simulink model "PHIL_DHS_XY_Control"  (R2019b)
settings: Solver=VariableStepAuto  StartTime=0.0  StopTime=00.2  RelTol=1e-3
undefined symbols (not defined in the file): Apd_i_dhs, Apd_u_dhs, C_dhs, f_sw_dhs, L_dhs, L_drom, Tid_i_dhs, Tid_u_dhs, U_DC
libraries: coordinate_transformations x9, simulink x8
settings Model: Creator=kissd  LastModifiedBy=kissd

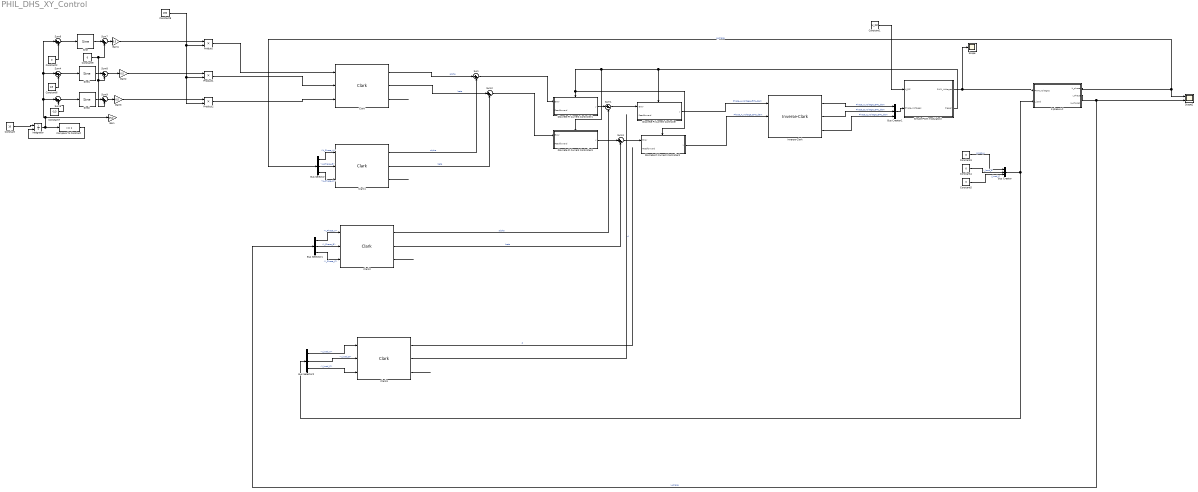
== system PHIL_DHS_XY_Control ==
  3 phase LC : Subsystem
  Bus Creator : BusCreator  Inputs=3
  Bus Creator1 : BusCreator  Inputs=3
  Bus Selector : BusSelector  OutputSignals=U_Phase_A,U_Phase_B,U_Phase_C
  Bus Selector1 : BusSelector  OutputSignals=I_Phase_A,I_Phase_B,I_Phase_C
  Bus Selector2 : BusSelector  OutputSignals=I_load_A,I_load_B,I_load_C
  Clark{,1..3} (4 alike) : coordinate_transformations/Clark  SystemSampleTime=-1  Latency=0  AutoFrameSizeCalculation=off
  Compare To Constant : simulink/Logic and Bit Operations/Compare To Constant  relop=>=  const=1  OutDataTypeStr=boolean
  Constant : Constant  Value=10
  Constant1 : Constant  Value=U_DC
  Constant{2..5,9} (5 alike) : Constant  Value=0
  Constant6 : Constant  Value=1/3
  Constant7 : Constant  Value=-1/3
  Constant8 : Constant  Value=200
  Discrete PI Current Controller : Subsystem  AncestorBlock=controllers/Discrete PI Controller  mask(Continous PI Controller){Apd=Apd_i_dhs, Tid=Tid_i_dhs, fs=f_sw_dhs, UpperSat=U_DC, LowerSat=0}
      mask prompts: Apd "Proprotional Gain"; Tid "Integration Time"; fs "fsw"; UpperSat "Max. Saturation"; LowerSat "Min. Saturation"
      mask help: Continous PI Controller description.
  Discrete PI Current Controller1 : Subsystem  AncestorBlock=controllers/Discrete PI Controller  mask(Continous PI Controller){Apd=Apd_u_dhs, Tid=Tid_u_dhs, fs=f_sw_dhs, UpperSat=200, LowerSat=-200}
      mask prompts: Apd "Proprotional Gain"; Tid "Integration Time"; fs "fsw"; UpperSat "Max. Saturation"; LowerSat "Min. Saturation"
      mask help: Continous PI Controller description.
  Discrete PI Current Controller2 : Subsystem  AncestorBlock=controllers/Discrete PI Controller  mask(Continous PI Controller){Apd=Apd_i_dhs, Tid=Tid_i_dhs, fs=f_sw_dhs, UpperSat=U_DC, LowerSat=0}
      mask prompts: Apd "Proprotional Gain"; Tid "Integration Time"; fs "fsw"; UpperSat "Max. Saturation"; LowerSat "Min. Saturation"
      mask help: Continous PI Controller description.
  Discrete PI Current Controller3 : Subsystem  AncestorBlock=controllers/Discrete PI Controller  mask(Continous PI Controller){Apd=Apd_u_dhs, Tid=Tid_u_dhs, fs=f_sw_dhs, UpperSat=200, LowerSat=-200}
      mask prompts: Apd "Proprotional Gain"; Tid "Integration Time"; fs "fsw"; UpperSat "Max. Saturation"; LowerSat "Min. Saturation"
      mask help: Continous PI Controller description.
  Gain : Gain  Gain=2*pi
  Gain1 : Gain  Gain=0.5
  Gain2 : Gain  Gain=0.5
  Gain3 : Gain  Gain=0.5
  Integrator : Integrator  ExternalReset=either
  Inverse-Clark : coordinate_transformations/Inverse-Clark  SystemSampleTime=-1  Latency=0  AutoFrameSizeCalculation=off
  Product : Product
  Product1 : Product
  Product2 : Product
  Scope : Scope
  Scope2 : Scope  NumInputPorts=2
  Simple PWM modulator2 : Subsystem  AncestorBlock=controllers/Simple PWM modulator
  Sine : simulink/Lookup Tables/Sine  Formula=sin(2*pi*u)  NumDataPoints=(2^5)+1  OutputWordLength=16  InternalRulePriority=Speed
      settings: SourceProductName=Simulink
  Sine1 : simulink/Lookup Tables/Sine  Formula=sin(2*pi*u)  NumDataPoints=(2^5)+1  OutputWordLength=16  InternalRulePriority=Speed
      settings: SourceProductName=Simulink
  Sine2 : simulink/Lookup Tables/Sine  Formula=sin(2*pi*u)  NumDataPoints=(2^5)+1  OutputWordLength=16  InternalRulePriority=Speed
      settings: SourceProductName=Simulink
  Sum{,1..3} (4 alike) : Sum  Inputs=|+-
  Sum{4..9} (6 alike) : Sum  Inputs=|++
  wires:
  Constant1/1 -> Simple PWM modulator2/1(U_DC)
  Inverse-Clark/3 -> Bus Creator1/3  "Phase_C_Voltage_EMU_dem"
  Inverse-Clark/2 -> Bus Creator1/2  "Phase_B_Voltage_EMU_dem"
  Sum1/1 -> Discrete PI Current Controller/1(Error)
  Inverse-Clark/1 -> Bus Creator1/1  "Phase_A_Voltage_EMU_dem"
  Simple PWM modulator2/1(PWM_Voltages) -> Scope/1, 3 phase LC/1(PWM_Voltages)
  Bus Creator1/1 -> Simple PWM modulator2/2(Phase_Voltages)
  Discrete PI Current Controller1/1(y) -> Sum1/1
  Sum/1 -> Discrete PI Current Controller1/1(Error)
  Clark/1 -> Sum/1  "alpha"
  Clark/2 -> Sum2/1  "beta"
  Clark/3 -> ?
  3 phase LC/2(I_Phase) -> Bus Selector1/1, Scope2/2  "I_phase"
  3 phase LC/1(U_phase) -> Scope2/1, Bus Selector/1  "U_phase"
  Constant3/1 -> Bus Creator/1  "I_load_A"
  Constant4/1 -> Bus Creator/2  "I_load_B"
  Constant5/1 -> Bus Creator/3  "I_load_C"
  Bus Creator/1 -> Bus Selector2/1, 3 phase LC/2(I_load)
  Discrete PI Current Controller/1(y) -> Inverse-Clark/1  "Phase_A_Voltage_EMU_dem"
  Sum2/1 -> Discrete PI Current Controller3/1(Error)
  Discrete PI Current Controller3/1(y) -> Sum3/1
  Sum3/1 -> Discrete PI Current Controller2/1(Error)
  Discrete PI Current Controller2/1(y) -> Inverse-Clark/2  "Phase_A_Voltage_EMU_dem"
  Clark1/3 -> ?
  Clark1/1 -> Sum/2  "alpha"
  Clark1/2 -> Sum2/2  "beta"
  Clark2/3 -> ?
  Bus Selector/1 -> Clark1/1  "<U_Phase_A>"
  Bus Selector/2 -> Clark1/2  "<U_Phase_B>"
  Bus Selector/3 -> Clark1/3  "<U_Phase_C>"
  Bus Selector1/1 -> Clark2/1  "<I_Phase_A>"
  Bus Selector1/2 -> Clark2/2  "<I_Phase_B>"
  Bus Selector1/3 -> Clark2/3  "<I_Phase_C>"
  Clark2/1 -> Sum1/2  "alpha"
  Clark2/2 -> Sum3/2  "beta"
  Bus Selector2/3 -> Clark3/3  "<I_load_C>"
  Bus Selector2/1 -> Clark3/1  "<I_load_A>"
  Clark3/3 -> ?
  Bus Selector2/2 -> Clark3/2  "<I_load_B>"
  Clark3/1 -> ?  "d"
  Clark3/2 -> ?  "d"
  Simple PWM modulator2/2(trigger) -> Discrete PI Current Controller2/Trigger, Discrete PI Current Controller1/Trigger, Discrete PI Current Controller3/Trigger, Discrete PI Current Controller/Trigger
  Sum4/1 -> Sine1/1
  Sum5/1 -> Sine2/1
  Sum6/1 -> Sine/1
  Constant/1 -> Integrator/1
  Compare To Constant/1 -> Integrator/2
  Constant2/1 -> Sum6/2
  Constant6/1 -> Sum4/2
  Constant7/1 -> Sum5/2
  Sine/1 -> Sum7/1
  Integrator/1 -> Gain/1, Sum5/1, Sum4/1, Sum6/1, Compare To Constant/1
  Constant8/1 -> Product2/2, Product1/2, Product/2
  Product/1 -> Clark/1
  Product1/1 -> Clark/2
  Product2/1 -> Clark/3
  Sine1/1 -> Sum8/1
  Sine2/1 -> Sum9/1
  Sum9/1 -> Gain3/1
  Sum8/1 -> Gain2/1
  Sum7/1 -> Gain1/1
  Constant9/1 -> Sum7/2, Sum8/2, Sum9/2
  Gain1/1 -> Product/1
  Gain2/1 -> Product1/1
  Gain3/1 -> Product2/1

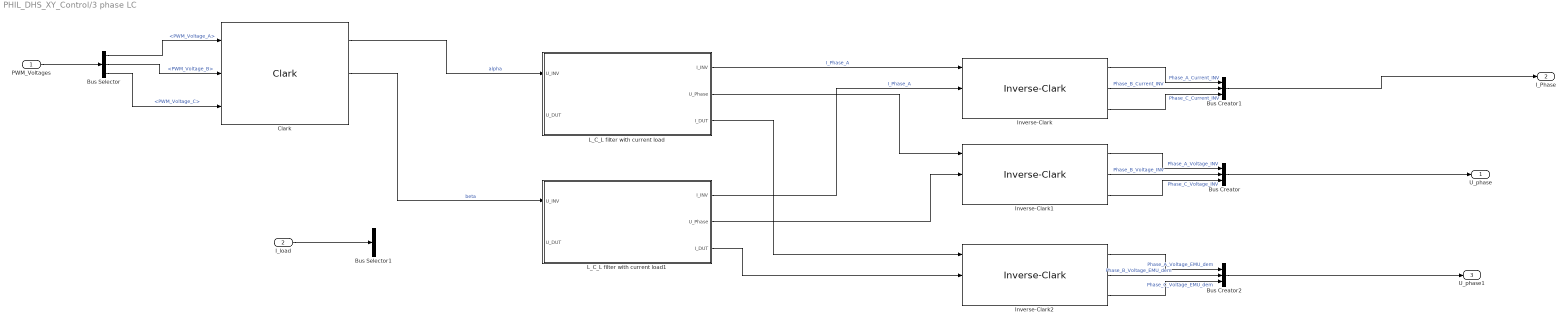
== system PHIL_DHS_XY_Control/3 phase LC ==
  PWM_Voltages : Inport
  I_load : Inport  Port=2
  Bus Creator : BusCreator  Inputs=3
  Bus Creator1 : BusCreator  Inputs=3
  Bus Creator2 : BusCreator  Inputs=3
  Bus Selector : BusSelector  OutputSignals=PWM_Voltage_A,PWM_Voltage_B,PWM_Voltage_C
  Bus Selector1 : BusSelector  OutputSignals=I_load_A,I_load_B,I_load_C
  Clark : coordinate_transformations/Clark  SystemSampleTime=-1  Latency=0  AutoFrameSizeCalculation=off
  Inverse-Clark : coordinate_transformations/Inverse-Clark  SystemSampleTime=-1  Latency=0  AutoFrameSizeCalculation=off
  Inverse-Clark1 : coordinate_transformations/Inverse-Clark  SystemSampleTime=-1  Latency=0  AutoFrameSizeCalculation=off
  Inverse-Clark2 : coordinate_transformations/Inverse-Clark  SystemSampleTime=-1  Latency=0  AutoFrameSizeCalculation=off
  L_C_L filter with current load : Subsystem
  L_C_L filter with current load1 : Subsystem
  U_phase : Outport
  I_Phase : Outport  Port=2
  U_phase1 : Outport  Port=3
  wires:
  PWM_Voltages/1 -> Bus Selector/1
  Bus Creator/1 -> U_phase/1
  Bus Creator1/1 -> I_Phase/1
  I_load/1 -> Bus Selector1/1
  Bus Selector/2 -> Clark/2  "<PWM_Voltage_B>"
  Bus Selector/1 -> Clark/1  "<PWM_Voltage_A>"
  Bus Selector/3 -> Clark/3  "<PWM_Voltage_C>"
  Clark/1 -> L_C_L filter with current load/1(U_INV)  "alpha"
  Clark/2 -> L_C_L filter with current load1/1(U_INV)  "beta"
  L_C_L filter with current load/1(I_INV) -> Inverse-Clark/1  "I_Phase_A"
  L_C_L filter with current load1/1(I_INV) -> Inverse-Clark/2  "I_Phase_A"
  L_C_L filter with current load/2(U_Phase) -> Inverse-Clark1/1
  L_C_L filter with current load1/2(U_Phase) -> Inverse-Clark1/2
  L_C_L filter with current load/3(I_DUT) -> Inverse-Clark2/1
  L_C_L filter with current load1/3(I_DUT) -> Inverse-Clark2/2
  Inverse-Clark1/2 -> Bus Creator/2  "Phase_B_Voltage_INV"
  Inverse-Clark1/1 -> Bus Creator/1  "Phase_A_Voltage_INV"
  Inverse-Clark1/3 -> Bus Creator/3  "Phase_C_Voltage_INV"
  Inverse-Clark/2 -> Bus Creator1/2  "Phase_B_Current_INV"
  Inverse-Clark/1 -> Bus Creator1/1  "Phase_A_Current_INV"
  Inverse-Clark/3 -> Bus Creator1/3  "Phase_C_Current_INV"
  Inverse-Clark2/1 -> Bus Creator2/1  "Phase_A_Voltage_EMU_dem"
  Inverse-Clark2/2 -> Bus Creator2/2  "Phase_B_Voltage_EMU_dem"
  Inverse-Clark2/3 -> Bus Creator2/3  "Phase_C_Voltage_EMU_dem"
  Bus Creator2/1 -> U_phase1/1

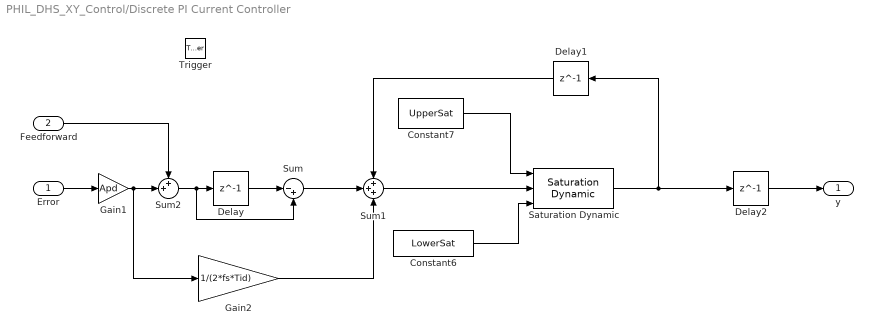
== system PHIL_DHS_XY_Control/Discrete PI Current Controller ==
  Error : Inport
  Feedforward : Inport  Port=2
  Trigger : TriggerPort  TriggerType=either  VariantControl=Variant  PortDimensions=1
  Constant6 : Constant  Value=LowerSat
  Constant7 : Constant  Value=UpperSat
  Delay : Delay  DelayLength=1
  Delay1 : Delay  DelayLength=1
  Delay2 : Delay  DelayLength=1
  Gain1 : Gain  Gain=Apd
  Gain2 : Gain  Gain=1/(2*fs*Tid)
  Saturation Dynamic : simulink/Discontinuities/Saturation Dynamic  OutMin=[]  OutMax=[]  OutDataTypeStr=Inherit: Same as second input  OutDataType=fixdt(1, 16)  OutScaling=2^-10  DoSatur=off
  Sum : Sum  Inputs=|-+
  Sum1 : Sum  Inputs=+++
  Sum2 : Sum  Inputs=++|
  y : Outport
  wires:
  Error/1 -> Gain1/1
  Gain1/1 -> Sum2/2, Gain2/1
  Sum1/1 -> Saturation Dynamic/2
  Saturation Dynamic/1 -> Delay1/1, Delay2/1
  Constant7/1 -> Saturation Dynamic/1
  Constant6/1 -> Saturation Dynamic/3
  Delay/1 -> Sum/1
  Sum/1 -> Sum1/2
  Gain2/1 -> Sum1/3
  Delay1/1 -> Sum1/1
  Delay2/1 -> y/1
  Sum2/1 -> Sum/2, Delay/1
  Feedforward/1 -> Sum2/1

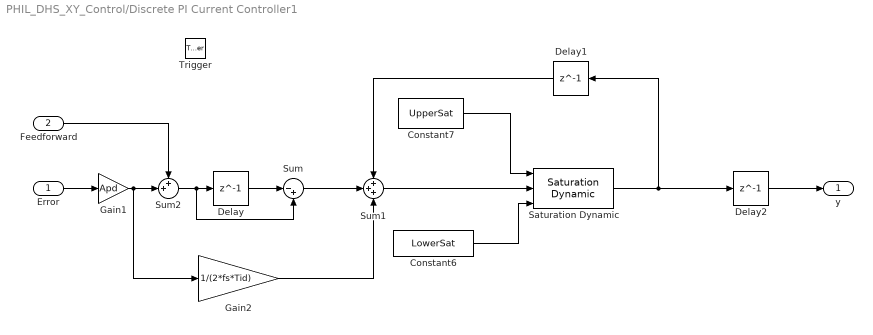
== system PHIL_DHS_XY_Control/Discrete PI Current Controller1 ==
  Error : Inport
  Feedforward : Inport  Port=2
  Trigger : TriggerPort  TriggerType=either  VariantControl=Variant  PortDimensions=1
  Constant6 : Constant  Value=LowerSat
  Constant7 : Constant  Value=UpperSat
  Delay : Delay  DelayLength=1
  Delay1 : Delay  DelayLength=1
  Delay2 : Delay  DelayLength=1
  Gain1 : Gain  Gain=Apd
  Gain2 : Gain  Gain=1/(2*fs*Tid)
  Saturation Dynamic : simulink/Discontinuities/Saturation Dynamic  OutMin=[]  OutMax=[]  OutDataTypeStr=Inherit: Same as second input  OutDataType=fixdt(1, 16)  OutScaling=2^-10  DoSatur=off
  Sum : Sum  Inputs=|-+
  Sum1 : Sum  Inputs=+++
  Sum2 : Sum  Inputs=++|
  y : Outport
  wires:
  Error/1 -> Gain1/1
  Gain1/1 -> Sum2/2, Gain2/1
  Sum1/1 -> Saturation Dynamic/2
  Saturation Dynamic/1 -> Delay1/1, Delay2/1
  Constant7/1 -> Saturation Dynamic/1
  Constant6/1 -> Saturation Dynamic/3
  Delay/1 -> Sum/1
  Sum/1 -> Sum1/2
  Gain2/1 -> Sum1/3
  Delay1/1 -> Sum1/1
  Delay2/1 -> y/1
  Sum2/1 -> Sum/2, Delay/1
  Feedforward/1 -> Sum2/1

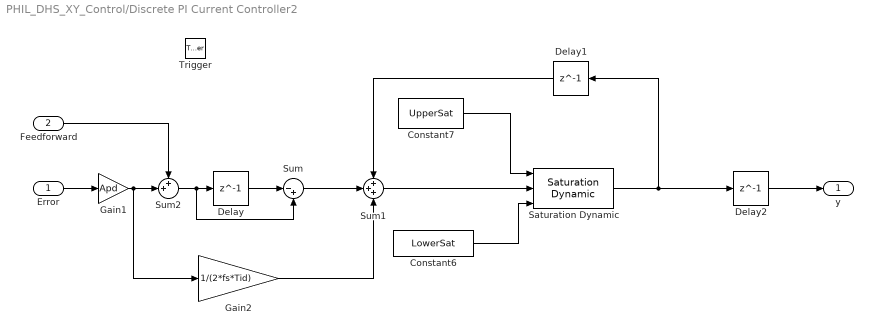
== system PHIL_DHS_XY_Control/Discrete PI Current Controller2 ==
  Error : Inport
  Feedforward : Inport  Port=2
  Trigger : TriggerPort  TriggerType=either  VariantControl=Variant  PortDimensions=1
  Constant6 : Constant  Value=LowerSat
  Constant7 : Constant  Value=UpperSat
  Delay : Delay  DelayLength=1
  Delay1 : Delay  DelayLength=1
  Delay2 : Delay  DelayLength=1
  Gain1 : Gain  Gain=Apd
  Gain2 : Gain  Gain=1/(2*fs*Tid)
  Saturation Dynamic : simulink/Discontinuities/Saturation Dynamic  OutMin=[]  OutMax=[]  OutDataTypeStr=Inherit: Same as second input  OutDataType=fixdt(1, 16)  OutScaling=2^-10  DoSatur=off
  Sum : Sum  Inputs=|-+
  Sum1 : Sum  Inputs=+++
  Sum2 : Sum  Inputs=++|
  y : Outport
  wires:
  Error/1 -> Gain1/1
  Gain1/1 -> Sum2/2, Gain2/1
  Sum1/1 -> Saturation Dynamic/2
  Saturation Dynamic/1 -> Delay1/1, Delay2/1
  Constant7/1 -> Saturation Dynamic/1
  Constant6/1 -> Saturation Dynamic/3
  Delay/1 -> Sum/1
  Sum/1 -> Sum1/2
  Gain2/1 -> Sum1/3
  Delay1/1 -> Sum1/1
  Delay2/1 -> y/1
  Sum2/1 -> Sum/2, Delay/1
  Feedforward/1 -> Sum2/1

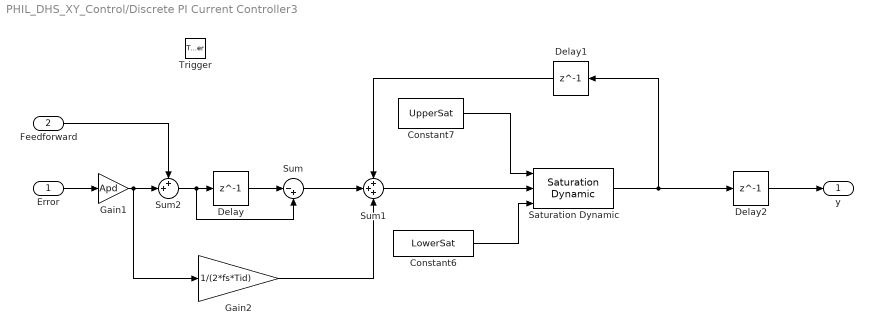
== system PHIL_DHS_XY_Control/Discrete PI Current Controller3 ==
  Error : Inport
  Feedforward : Inport  Port=2
  Trigger : TriggerPort  TriggerType=either  VariantControl=Variant  PortDimensions=1
  Constant6 : Constant  Value=LowerSat
  Constant7 : Constant  Value=UpperSat
  Delay : Delay  DelayLength=1
  Delay1 : Delay  DelayLength=1
  Delay2 : Delay  DelayLength=1
  Gain1 : Gain  Gain=Apd
  Gain2 : Gain  Gain=1/(2*fs*Tid)
  Saturation Dynamic : simulink/Discontinuities/Saturation Dynamic  OutMin=[]  OutMax=[]  OutDataTypeStr=Inherit: Same as second input  OutDataType=fixdt(1, 16)  OutScaling=2^-10  DoSatur=off
  Sum : Sum  Inputs=|-+
  Sum1 : Sum  Inputs=+++
  Sum2 : Sum  Inputs=++|
  y : Outport
  wires:
  Error/1 -> Gain1/1
  Gain1/1 -> Sum2/2, Gain2/1
  Sum1/1 -> Saturation Dynamic/2
  Saturation Dynamic/1 -> Delay1/1, Delay2/1
  Constant7/1 -> Saturation Dynamic/1
  Constant6/1 -> Saturation Dynamic/3
  Delay/1 -> Sum/1
  Sum/1 -> Sum1/2
  Gain2/1 -> Sum1/3
  Delay1/1 -> Sum1/1
  Delay2/1 -> y/1
  Sum2/1 -> Sum/2, Delay/1
  Feedforward/1 -> Sum2/1

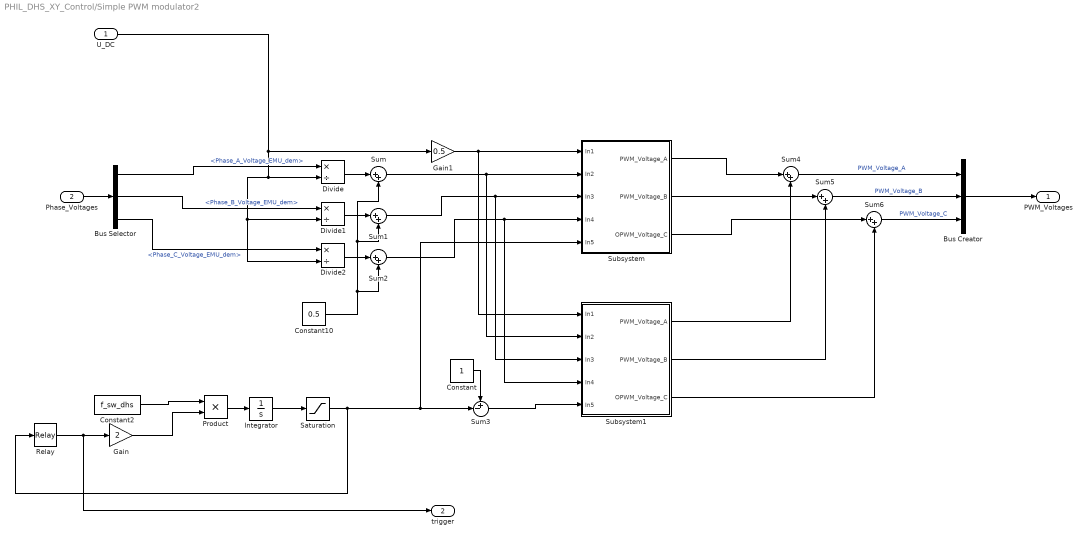
== system PHIL_DHS_XY_Control/Simple PWM modulator2 ==
  U_DC : Inport
  Phase_Voltages : Inport  Port=2
  Bus Creator : BusCreator  Inputs=3
  Bus Selector : BusSelector  OutputSignals=Phase_A_Voltage_EMU_dem,Phase_B_Voltage_EMU_dem,Phase_C_Voltage_EMU_dem
  Constant : Constant
  Constant10 : Constant  Value=0.5
  Constant2 : Constant  Value=f_sw_dhs
  Divide : Product  Inputs=*/
  Divide1 : Product  Inputs=*/
  Divide2 : Product  Inputs=*/
  Gain : Gain  Gain=2
  Gain1 : Gain  Gain=0.5
  Integrator : Integrator
  Product : Product
  Relay : Relay  OnSwitchValue=1  OffSwitchValue=0  OnOutputValue=-1  OffOutputValue=1
  Saturation : Saturate  UpperLimit=1  LowerLimit=0
  Subsystem : Subsystem
  Subsystem1 : Subsystem
  Sum{,1..2,4..6} (6 alike) : Sum  Inputs=|++
  Sum3 : Sum  Inputs=+-|
  PWM_Voltages : Outport
  trigger : Outport  Port=2
  wires:
  Constant2/1 -> Product/1
  Product/1 -> Integrator/1
  Integrator/1 -> Saturation/1
  Divide1/1 -> Sum1/1
  Saturation/1 -> Subsystem/5(In5), Sum3/2, Relay/1
  Relay/1 -> trigger/1, Gain/1
  Constant10/1 -> Sum2/2, Sum1/2, Sum/2
  Bus Selector/1 -> Divide/1  "<Phase_A_Voltage_EMU_dem>"
  Gain/1 -> Product/2
  Divide2/1 -> Sum2/1
  Divide/1 -> Sum/1
  Bus Selector/3 -> Divide2/1  "<Phase_C_Voltage_EMU_dem>"
  Bus Selector/2 -> Divide1/1  "<Phase_B_Voltage_EMU_dem>"
  Phase_Voltages/1 -> Bus Selector/1
  Bus Creator/1 -> PWM_Voltages/1
  Constant/1 -> Sum3/1
  Sum/1 -> Subsystem1/2(In2), Subsystem/2(In2)
  Sum1/1 -> Subsystem1/3(In3), Subsystem/3(In3)
  Sum2/1 -> Subsystem1/4(In4), Subsystem/4(In4)
  Sum3/1 -> Subsystem1/5(In5)
  Sum4/1 -> Bus Creator/1  "PWM_Voltage_A"
  Subsystem/1(PWM_Voltage_A) -> Sum4/1
  Subsystem1/1(PWM_Voltage_A) -> Sum4/2
  Sum5/1 -> Bus Creator/2  "PWM_Voltage_B"
  Subsystem/2(PWM_Voltage_B) -> Sum5/1
  Subsystem1/2(PWM_Voltage_B) -> Sum5/2
  Sum6/1 -> Bus Creator/3  "PWM_Voltage_C"
  Subsystem/3(OPWM_Voltage_C) -> Sum6/1
  Subsystem1/3(OPWM_Voltage_C) -> Sum6/2
  U_DC/1 -> Gain1/1, Divide2/2, Divide1/2, Divide/2
  Gain1/1 -> Subsystem1/1(In1), Subsystem/1(In1)

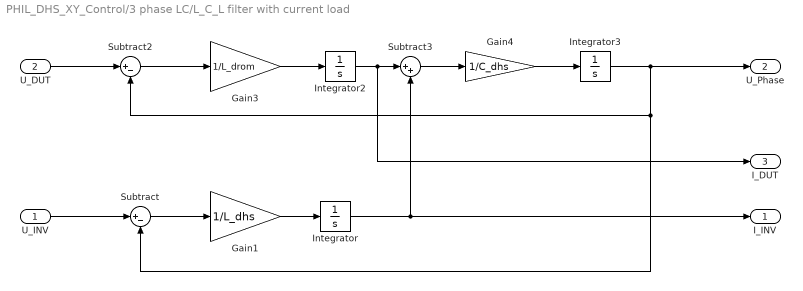
== system PHIL_DHS_XY_Control/3 phase LC/L_C_L filter with current load ==
  U_INV : Inport
  U_DUT : Inport  Port=2
  Gain1 : Gain  Gain=1/L_dhs
  Gain3 : Gain  Gain=1/L_drom
  Gain4 : Gain  Gain=1/C_dhs
  Integrator : Integrator
  Integrator2 : Integrator
  Integrator3 : Integrator
  Subtract : Sum  Inputs=|+-
  Subtract2 : Sum  Inputs=|+-
  Subtract3 : Sum  Inputs=|++
  I_INV : Outport
  U_Phase : Outport  Port=2
  I_DUT : Outport  Port=3
  wires:
  Subtract/1 -> Gain1/1
  Gain1/1 -> Integrator/1
  Integrator/1 -> Subtract3/2, I_INV/1
  U_INV/1 -> Subtract/1
  U_DUT/1 -> Subtract2/1
  Subtract2/1 -> Gain3/1
  Gain3/1 -> Integrator2/1
  Integrator2/1 -> I_DUT/1, Subtract3/1
  Subtract3/1 -> Gain4/1
  Gain4/1 -> Integrator3/1
  Integrator3/1 -> Subtract2/2, Subtract/2, U_Phase/1

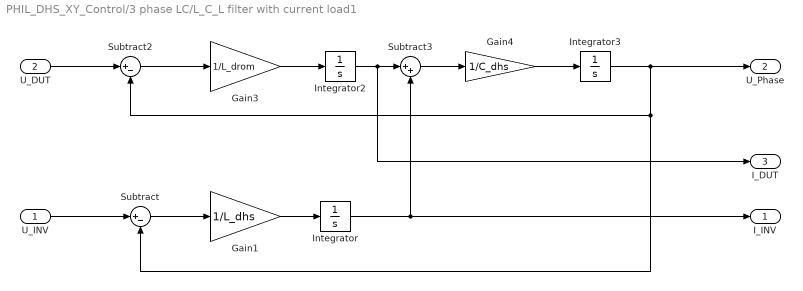
== system PHIL_DHS_XY_Control/3 phase LC/L_C_L filter with current load1 ==
  U_INV : Inport
  U_DUT : Inport  Port=2
  Gain1 : Gain  Gain=1/L_dhs
  Gain3 : Gain  Gain=1/L_drom
  Gain4 : Gain  Gain=1/C_dhs
  Integrator : Integrator
  Integrator2 : Integrator
  Integrator3 : Integrator
  Subtract : Sum  Inputs=|+-
  Subtract2 : Sum  Inputs=|+-
  Subtract3 : Sum  Inputs=|++
  I_INV : Outport
  U_Phase : Outport  Port=2
  I_DUT : Outport  Port=3
  wires:
  Subtract/1 -> Gain1/1
  Gain1/1 -> Integrator/1
  Integrator/1 -> Subtract3/2, I_INV/1
  U_INV/1 -> Subtract/1
  U_DUT/1 -> Subtract2/1
  Subtract2/1 -> Gain3/1
  Gain3/1 -> Integrator2/1
  Integrator2/1 -> I_DUT/1, Subtract3/1
  Subtract3/1 -> Gain4/1
  Gain4/1 -> Integrator3/1
  Integrator3/1 -> Subtract2/2, Subtract/2, U_Phase/1

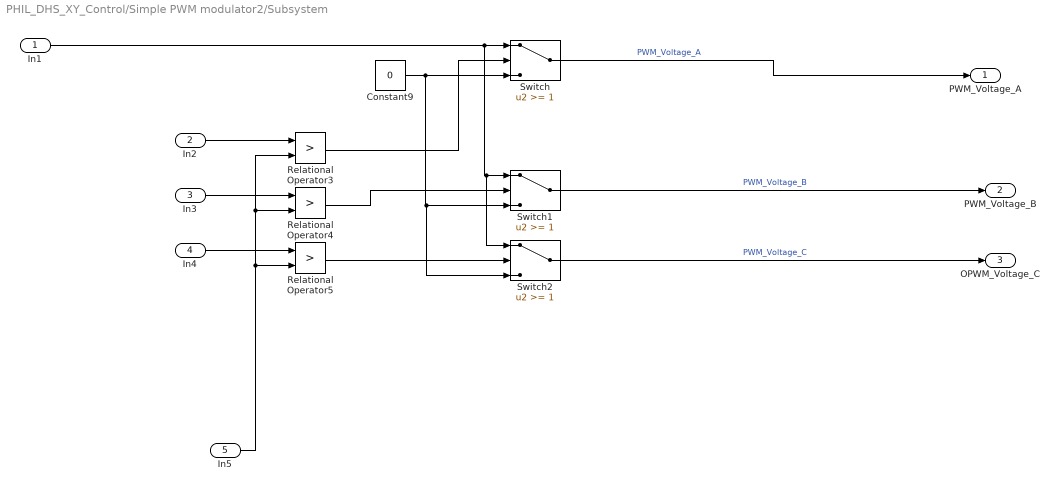
== system PHIL_DHS_XY_Control/Simple PWM modulator2/Subsystem ==
  In1 : Inport
  In2 : Inport  Port=2
  In3 : Inport  Port=3
  In4 : Inport  Port=4
  In5 : Inport  Port=5
  Constant9 : Constant  Value=0
  Relational Operator3 : RelationalOperator  Operator=>  OutDataTypeStr=boolean  RndMeth=Simplest
  Relational Operator4 : RelationalOperator  Operator=>  OutDataTypeStr=boolean  RndMeth=Simplest
  Relational Operator5 : RelationalOperator  Operator=>  OutDataTypeStr=boolean  RndMeth=Simplest
  Switch : Switch  Threshold=1
  Switch1 : Switch  Threshold=1
  Switch2 : Switch  Threshold=1
  PWM_Voltage_A : Outport
  PWM_Voltage_B : Outport  Port=2
  OPWM_Voltage_C : Outport  Port=3
  wires:
  Relational Operator4/1 -> Switch1/2
  In5/1 -> Relational Operator3/2, Relational Operator4/2, Relational Operator5/2
  Constant9/1 -> Switch2/3, Switch1/3, Switch/3
  Relational Operator3/1 -> Switch/2
  In3/1 -> Relational Operator4/1
  Relational Operator5/1 -> Switch2/2
  Switch/1 -> PWM_Voltage_A/1  "PWM_Voltage_A"
  In1/1 -> Switch2/1, Switch1/1, Switch/1
  In2/1 -> Relational Operator3/1
  In4/1 -> Relational Operator5/1
  Switch1/1 -> PWM_Voltage_B/1  "PWM_Voltage_B"
  Switch2/1 -> OPWM_Voltage_C/1  "PWM_Voltage_C"

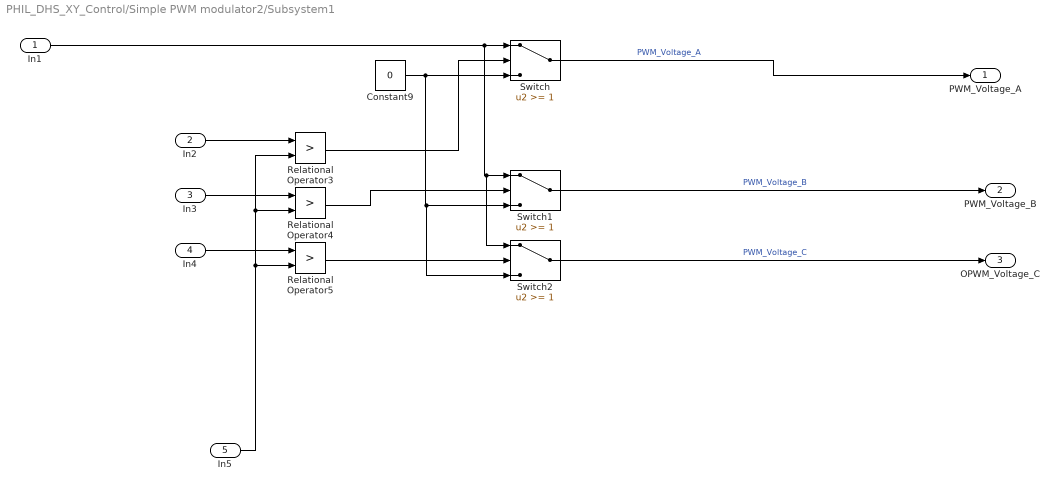
== system PHIL_DHS_XY_Control/Simple PWM modulator2/Subsystem1 ==
  In1 : Inport
  In2 : Inport  Port=2
  In3 : Inport  Port=3
  In4 : Inport  Port=4
  In5 : Inport  Port=5
  Constant9 : Constant  Value=0
  Relational Operator3 : RelationalOperator  Operator=>  OutDataTypeStr=boolean  RndMeth=Simplest
  Relational Operator4 : RelationalOperator  Operator=>  OutDataTypeStr=boolean  RndMeth=Simplest
  Relational Operator5 : RelationalOperator  Operator=>  OutDataTypeStr=boolean  RndMeth=Simplest
  Switch : Switch  Threshold=1
  Switch1 : Switch  Threshold=1
  Switch2 : Switch  Threshold=1
  PWM_Voltage_A : Outport
  PWM_Voltage_B : Outport  Port=2
  OPWM_Voltage_C : Outport  Port=3
  wires:
  Relational Operator4/1 -> Switch1/2
  In5/1 -> Relational Operator3/2, Relational Operator4/2, Relational Operator5/2
  Constant9/1 -> Switch2/3, Switch1/3, Switch/3
  Relational Operator3/1 -> Switch/2
  In3/1 -> Relational Operator4/1
  Relational Operator5/1 -> Switch2/2
  Switch/1 -> PWM_Voltage_A/1  "PWM_Voltage_A"
  In1/1 -> Switch2/1, Switch1/1, Switch/1
  In2/1 -> Relational Operator3/1
  In4/1 -> Relational Operator5/1
  Switch1/1 -> PWM_Voltage_B/1  "PWM_Voltage_B"
  Switch2/1 -> OPWM_Voltage_C/1  "PWM_Voltage_C"
